simulink model "firststatespace"  (R2015a)
settings: Solver=ode45  StartTime=0.0  StopTime=10.0  RelTol=1e-3
values from neighbouring files (symbols this model uses):
  C = [0 1 0 0 0]    [Modeling2_6_5_2015.m]
  h = 0.05    [Modeling2_6_5_2015.m]
  K0d = inv(Cd*inv(eye(5)-Ad+Bd*Kd)*Bd)    [Modeling2_6_5_2015.m]
  Kd = place(Ad,Bd,Ppd)    [Modeling2_6_5_2015.m]
  Ld = (place(Ad',Cd',PpLD))'    [Modeling2_6_5_2015.m]
  workpoint = [0,0,0,0,0]    [Modeling2_6_5_2015.m]
undefined symbols (not defined in the file or in its folder): Ad, Bd, Cd, Model
settings Model: CovSFcnEnable=off  Creator=ovillarrealmag  LastModifiedBy=Tavo
settings DebuggingCC: SolverPrmCheckMsg=warning

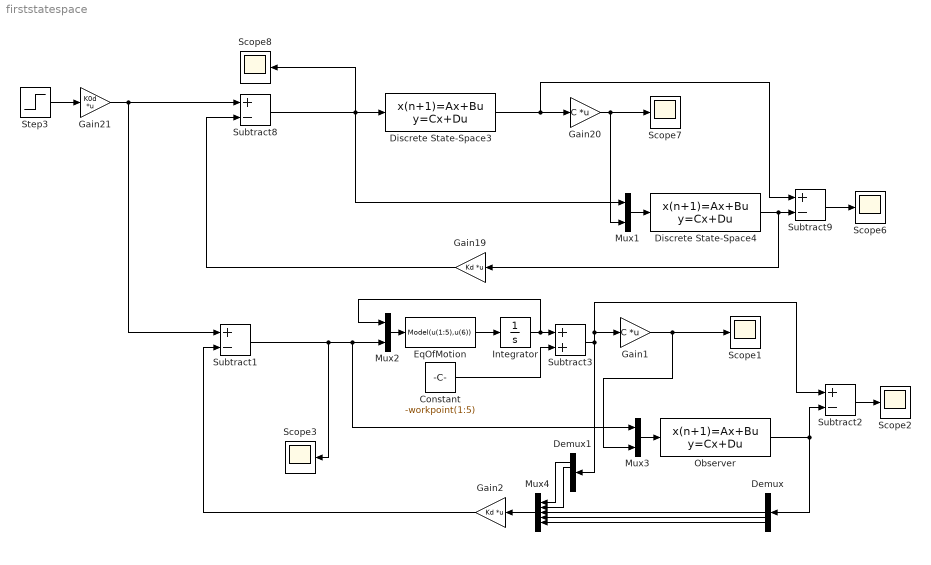
== system firststatespace ==
  Constant : Constant  Value=-workpoint(1:5)
  Demux : Demux  Outputs=5
  Demux1 : Demux  Outputs=5
  Discrete State-Space3 : DiscreteStateSpace  A=Ad  B=Bd  C=eye(5)  D=zeros(5,1)  X0=[0 0.1 0 0 0]  SampleTime=h
  Discrete State-Space4 : DiscreteStateSpace  A=Ad-Ld*Cd  B=[Bd Ld]  C=eye(5)  D=zeros(5,2)  SampleTime=h
  EqOfMotion : MATLABFcn  MATLABFcn=Model(u(1:5),u(6))  OutputDimensions=5
  Gain1 : Gain  Gain=C  Multiplication=Matrix(K*u)
  Gain19 : Gain  Gain=Kd  Multiplication=Matrix(K*u)
  Gain2 : Gain  Gain=Kd  Multiplication=Matrix(K*u)
  Gain20 : Gain  Gain=C  Multiplication=Matrix(K*u)
  Gain21 : Gain  Gain=K0d  Multiplication=Matrix(K*u)
  Integrator : Integrator  InitialCondition=workpoint(1:5) + [0 0.1 0 0 0]
  Mux1 : Mux  Inputs=2
  Mux2 : Mux  Inputs=2
  Mux3 : Mux  Inputs=2
  Mux4 : Mux  Inputs=5
  "Observer " : DiscreteStateSpace  A=Ad-Ld*Cd  B=[Bd Ld]  C=eye(5)  D=zeros(5,2)  X0=workpoint(1:5)  SampleTime=h
  Scope{1..3,6..8} (6 alike) : Scope
      Scope1 settings: YMin=-13000  YMax=-10500
      Scope2 settings: TimeRange=10  YMin=-2e+42  YMax=1.2e+43  SaveName=ScopeData3
      Scope3 settings: TimeRange=10  YMin=-2e+42  YMax=1.2e+43  SaveName=ScopeData4
      Scope6 settings: TimeRange=10  YMin=-2e+42  YMax=1.2e+43
      Scope7 settings: SaveName=ScopeData2
      Scope8 settings: TimeRange=10  YMin=-90  YMax=10  SaveName=outobs
  Step3 : Step  Time=0  After=0  SampleTime=0
  Subtract{1..2,8..9} (4 alike) : Sum  Inputs=+-
  Subtract3 : Sum
  wires:
  Step3/1 -> Gain21/1
  Subtract8/1 -> Discrete State-Space3/1, Mux1/1, Scope8/1
  Gain21/1 -> Subtract1/1, Subtract8/1
  Mux1/1 -> Discrete State-Space4/1
  Subtract9/1 -> Scope6/1
  Gain19/1 -> Subtract8/2
  Discrete State-Space3/1 -> Subtract9/1, Gain20/1
  Discrete State-Space4/1 -> Gain19/1, Subtract9/2
  Gain20/1 -> Scope7/1, Mux1/2
  Mux2/1 -> EqOfMotion/1
  EqOfMotion/1 -> Integrator/1
  Subtract1/1 -> Scope3/1, Mux3/1, Mux2/2
  Gain2/1 -> Subtract1/2
  Gain1/1 -> Scope1/1, Mux3/2
  Mux3/1 -> "Observer "/1
  Subtract2/1 -> Scope2/1
  "Observer "/1 -> Subtract2/2, Demux/1
  Demux/3 -> Mux4/3
  Demux/4 -> Mux4/4
  Mux4/1 -> Gain2/1
  Integrator/1 -> Mux2/1, Subtract3/1
  Constant/1 -> Subtract3/2
  Subtract3/1 -> Subtract2/1, Gain1/1, Demux1/1
  Demux1/1 -> Mux4/1
  Demux1/2 -> Mux4/2
  Demux/5 -> Mux4/5
